simulink model "SWC_OUTP_type"  (R2021b)
settings: Solver=FixedStepDiscrete  StartTime=0.0  StopTime=10.0  FixedStep=0.005  RelTol=1e-3
undefined symbols (not defined in the file): FALSE, TRUE
libraries: outp x1
settings Model: DataDictionary=APPTypes.sldd  Creator=FVT23010  LastModifiedBy=FVT23033
settings DataIOCC: SaveFormat=StructureWithTime
settings OptimizationCC: DefaultParameterBehavior=Inlined  EnhancedBackFolding=on  PassReuseOutputArgsAs=Individual arguments  ZeroExternalMemoryAtStartup=off  ZeroInternalMemoryAtStartup=off  OptimizeBlockOrder=speed  DifferentSizesBufferReuse=on  OptimizationCustomize=off  EfficientTunableParamExpr=on
settings DebuggingCC: ParameterTunabilityLossMsg=error
settings HardwareCC: ProdBitPerPointer=32  ProdBitPerSizeT=32  ProdBitPerPtrDiffT=32  ProdLargestAtomicInteger=Long  ProdLargestAtomicFloat=Double  ProdWordSize=32  ProdLongLongMode=on  ProdHWDeviceType=ARM Compatible->ARM Cortex-M
settings ModelReferenceCC: ModelReferenceNumInstancesAllowed=Single
settings SFSimCC: MATLABDynamicMemAlloc=off
settings RTWCC: Description=AUTOSAR  SystemTargetFile=autosar.tlc  GenCodeOnly=on  TemplateMakefile=ert_default_tmf  PortableWordSizes=on
settings CodeAppCC: ForceParamTrailComments=on  IgnoreCustomStorageClasses=off  OperatorAnnotations=on  SimulinkDataObjDesc=on  SFDataObjDesc=on  InsertBlockDesc=on
settings STFCustomTargetCC: TargetLangStandard=C99 (ISO)  UtilityFuncGeneration=Shared location  MultiwordLength=256  ParMdlRefBuildCompliant=on  CompOptLevelCompliant=on  IncludeMdlTerminateFcn=off  CombineOutputUpdateFcns=on  SuppressErrorStatus=on  ERTCustomFileBanners=on  SupportNonFinite=off  SupportComplex=off  SupportContinuousTime=off  SupportNonInlinedSFcns=off  RemoveResetFunc=on  MATLABClassNameForMDSCustomization=Simulink.SoftwareTarget.ERTCustomization  AutosarCompliant=on  GRTInterface=off  UseToolchainInfoCompliant=on  GenerateSharedConstants=off  LookupTableObjectStructAxisOrder=2,1,3,4,...  LUTObjectStructOrderEvenSpacing=Size,Table,Breakpoints  SystemTargetFile=autosar.tlc
settings ERTTargetCC: TargetLangStandard=C99 (ISO)  UtilityFuncGeneration=Shared location  ConcurrentExecutionCompliant=off  IncludeMdlTerminateFcn=off  SuppressErrorStatus=on  SupportNonFinite=off  SupportComplex=off  ModelStepFunctionPrototypeControlCompliant=off  CPPClassGenCompliant=off  AutosarCompliant=on  GenerateSharedConstants=off  LookupTableObjectStructAxisOrder=2,1,3,4,...  LUTObjectStructOrderEvenSpacing=Size,Table,Breakpoints  GenerateASAP2=on  InlinedParameterPlacement=NonHierarchical  ERTCustomFileTemplate=example_file_process.tlc  ConvertIfToSwitch=off  SuppressUnreachableDefaultCases=off  BooleanTrueId=true_MatlabRTW  BooleanFalseId=false_MatlabRTW

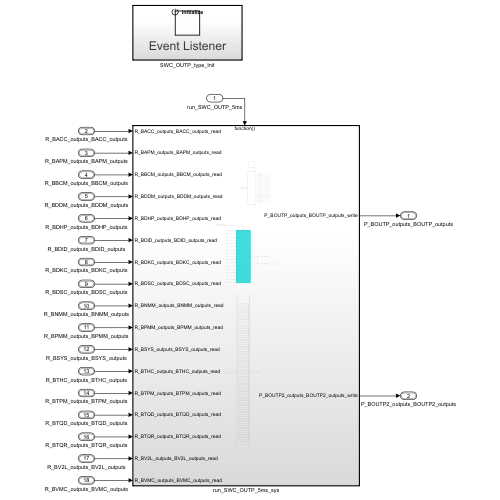
[thumbnail: Simulink's stored preview of the top-level diagram]
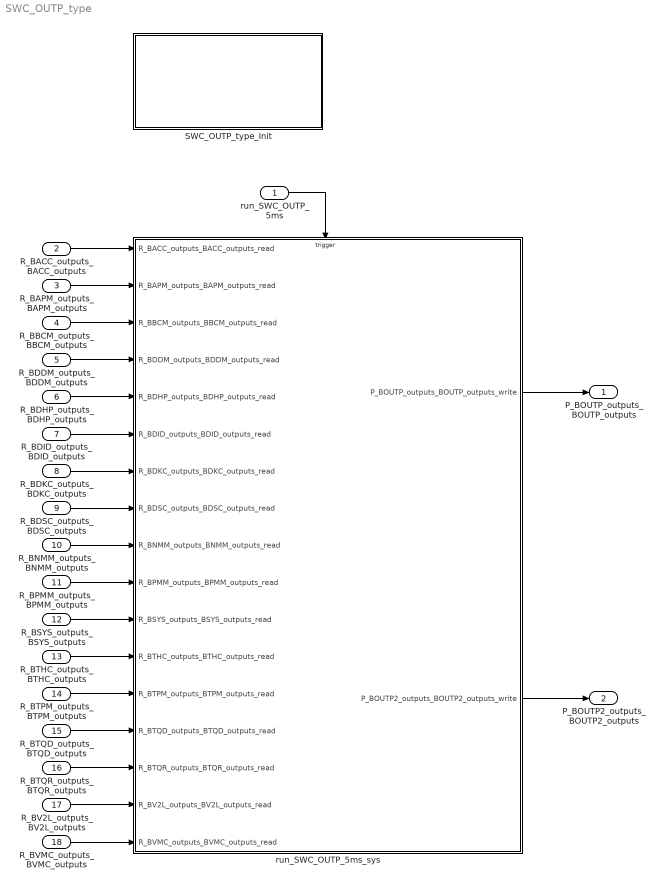
== system SWC_OUTP_type ==
  run_SWC_OUTP_5ms : Inport  SampleTime=0.005  OutputFunctionCall=on
  R_BACC_outputs_BACC_outputs : Inport  Port=2  OutDataTypeStr=Bus: BACC_outputs  PortDimensions=1  BusOutputAsStruct=on
  R_BAPM_outputs_BAPM_outputs : Inport  Port=3  OutDataTypeStr=Bus: BAPM_outputs  PortDimensions=1  BusOutputAsStruct=on
  R_BBCM_outputs_BBCM_outputs : Inport  Port=4  OutDataTypeStr=Bus: BBCM_outputs  PortDimensions=1  BusOutputAsStruct=on
  R_BDDM_outputs_BDDM_outputs : Inport  Port=5  OutDataTypeStr=Bus: BDDM_outputs  PortDimensions=1  BusOutputAsStruct=on
  R_BDHP_outputs_BDHP_outputs : Inport  Port=6  OutDataTypeStr=Bus: BDHP_outputs  PortDimensions=1  BusOutputAsStruct=on
  R_BDID_outputs_BDID_outputs : Inport  Port=7  OutDataTypeStr=Bus: BDID_outputs  PortDimensions=1  BusOutputAsStruct=on
  R_BDKC_outputs_BDKC_outputs : Inport  Port=8  OutDataTypeStr=Bus: BDKC_outputs  PortDimensions=1  BusOutputAsStruct=on
  R_BDSC_outputs_BDSC_outputs : Inport  Port=9  OutDataTypeStr=Bus: BDSC_outputs  PortDimensions=1  BusOutputAsStruct=on
  R_BNMM_outputs_BNMM_outputs : Inport  Port=10  OutDataTypeStr=Bus: BNMM_outputs  PortDimensions=1  BusOutputAsStruct=on
  R_BPMM_outputs_BPMM_outputs : Inport  Port=11  OutDataTypeStr=Bus: BPMM_outputs  PortDimensions=1  BusOutputAsStruct=on
  R_BSYS_outputs_BSYS_outputs : Inport  Port=12  OutDataTypeStr=Bus: BSYS_outputs  PortDimensions=1  BusOutputAsStruct=on
  R_BTHC_outputs_BTHC_outputs : Inport  Port=13  OutDataTypeStr=Bus: BTHC_outputs  PortDimensions=1  BusOutputAsStruct=on
  R_BTPM_outputs_BTPM_outputs : Inport  Port=14  OutDataTypeStr=Bus: BTPM_outputs  PortDimensions=1  BusOutputAsStruct=on
  R_BTQD_outputs_BTQD_outputs : Inport  Port=15  OutDataTypeStr=Bus: BTQD_outputs  PortDimensions=1  BusOutputAsStruct=on
  R_BTQR_outputs_BTQR_outputs : Inport  Port=16  OutDataTypeStr=Bus: BTQR_outputs  PortDimensions=1  BusOutputAsStruct=on
  R_BV2L_outputs_BV2L_outputs : Inport  Port=17  OutDataTypeStr=Bus: BV2L_outputs  PortDimensions=1  BusOutputAsStruct=on
  R_BVMC_outputs_BVMC_outputs : Inport  Port=18  OutDataTypeStr=Bus: BVMC_outputs  PortDimensions=1  BusOutputAsStruct=on
  SWC_OUTP_type_Init : Subsystem
  run_SWC_OUTP_5ms_sys : Subsystem
  P_BOUTP_outputs_BOUTP_outputs : Outport  OutDataTypeStr=Bus: BOUTP_outputs  PortDimensions=1  BusOutputAsStruct=on
  P_BOUTP2_outputs_BOUTP2_outputs : Outport  Port=2  OutDataTypeStr=Bus: BOUTP2_outputs  PortDimensions=1  BusOutputAsStruct=on
  wires:
  R_BACC_outputs_BACC_outputs/1 -> run_SWC_OUTP_5ms_sys/1(R_BACC_outputs_BACC_outputs_read)
  R_BAPM_outputs_BAPM_outputs/1 -> run_SWC_OUTP_5ms_sys/2(R_BAPM_outputs_BAPM_outputs_read)
  R_BBCM_outputs_BBCM_outputs/1 -> run_SWC_OUTP_5ms_sys/3(R_BBCM_outputs_BBCM_outputs_read)
  R_BDDM_outputs_BDDM_outputs/1 -> run_SWC_OUTP_5ms_sys/4(R_BDDM_outputs_BDDM_outputs_read)
  R_BDHP_outputs_BDHP_outputs/1 -> run_SWC_OUTP_5ms_sys/5(R_BDHP_outputs_BDHP_outputs_read)
  R_BDID_outputs_BDID_outputs/1 -> run_SWC_OUTP_5ms_sys/6(R_BDID_outputs_BDID_outputs_read)
  R_BDKC_outputs_BDKC_outputs/1 -> run_SWC_OUTP_5ms_sys/7(R_BDKC_outputs_BDKC_outputs_read)
  R_BDSC_outputs_BDSC_outputs/1 -> run_SWC_OUTP_5ms_sys/8(R_BDSC_outputs_BDSC_outputs_read)
  R_BNMM_outputs_BNMM_outputs/1 -> run_SWC_OUTP_5ms_sys/9(R_BNMM_outputs_BNMM_outputs_read)
  R_BPMM_outputs_BPMM_outputs/1 -> run_SWC_OUTP_5ms_sys/10(R_BPMM_outputs_BPMM_outputs_read)
  R_BSYS_outputs_BSYS_outputs/1 -> run_SWC_OUTP_5ms_sys/11(R_BSYS_outputs_BSYS_outputs_read)
  R_BTHC_outputs_BTHC_outputs/1 -> run_SWC_OUTP_5ms_sys/12(R_BTHC_outputs_BTHC_outputs_read)
  R_BTPM_outputs_BTPM_outputs/1 -> run_SWC_OUTP_5ms_sys/13(R_BTPM_outputs_BTPM_outputs_read)
  R_BTQD_outputs_BTQD_outputs/1 -> run_SWC_OUTP_5ms_sys/14(R_BTQD_outputs_BTQD_outputs_read)
  R_BTQR_outputs_BTQR_outputs/1 -> run_SWC_OUTP_5ms_sys/15(R_BTQR_outputs_BTQR_outputs_read)
  R_BV2L_outputs_BV2L_outputs/1 -> run_SWC_OUTP_5ms_sys/16(R_BV2L_outputs_BV2L_outputs_read)
  R_BVMC_outputs_BVMC_outputs/1 -> run_SWC_OUTP_5ms_sys/17(R_BVMC_outputs_BVMC_outputs_read)
  run_SWC_OUTP_5ms_sys/1(P_BOUTP_outputs_BOUTP_outputs_write) -> P_BOUTP_outputs_BOUTP_outputs/1
  run_SWC_OUTP_5ms_sys/2(P_BOUTP2_outputs_BOUTP2_outputs_write) -> P_BOUTP2_outputs_BOUTP2_outputs/1
  run_SWC_OUTP_5ms/1 -> run_SWC_OUTP_5ms_sys/Trigger

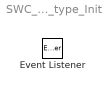
== system SWC_OUTP_type/SWC_OUTP_type_Init ==
  Event Listener : EventListener  EventName=reset

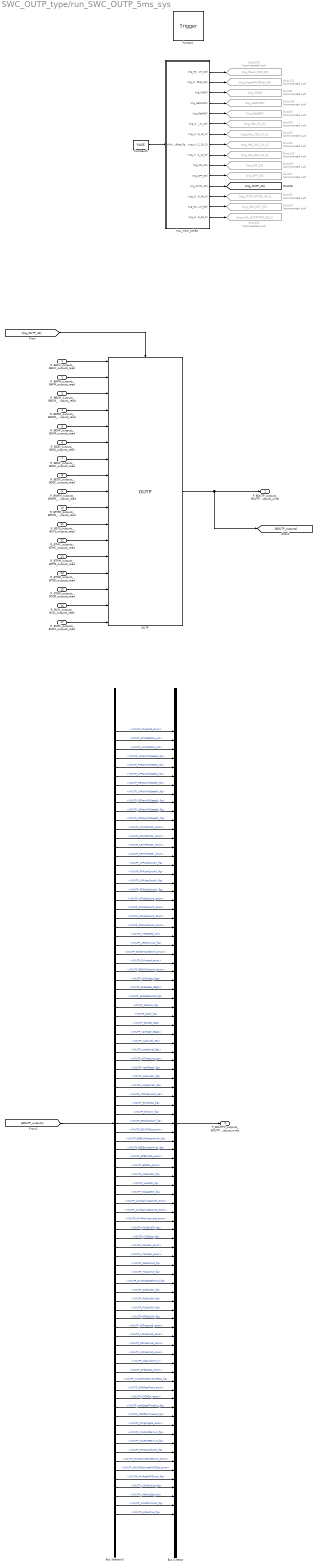
== system SWC_OUTP_type/run_SWC_OUTP_5ms_sys ==
  R_BACC_outputs_BACC_outputs_read : Inport
  R_BAPM_outputs_BAPM_outputs_read : Inport  Port=2
  R_BBCM_outputs_BBCM_outputs_read : Inport  Port=3
  R_BDDM_outputs_BDDM_outputs_read : Inport  Port=4
  R_BDHP_outputs_BDHP_outputs_read : Inport  Port=5
  R_BDID_outputs_BDID_outputs_read : Inport  Port=6
  R_BDKC_outputs_BDKC_outputs_read : Inport  Port=7
  R_BDSC_outputs_BDSC_outputs_read : Inport  Port=8
  R_BNMM_outputs_BNMM_outputs_read : Inport  Port=9
  R_BPMM_outputs_BPMM_outputs_read : Inport  Port=10
  R_BSYS_outputs_BSYS_outputs_read : Inport  Port=11
  R_BTHC_outputs_BTHC_outputs_read : Inport  Port=12
  R_BTPM_outputs_BTPM_outputs_read : Inport  Port=13
  R_BTQD_outputs_BTQD_outputs_read : Inport  Port=14
  R_BTQR_outputs_BTQR_outputs_read : Inport  Port=15
  R_BV2L_outputs_BV2L_outputs_read : Inport  Port=16
  R_BVMC_outputs_BVMC_outputs_read : Inport  Port=17
  function : TriggerPort  TriggerType=function-call  VariantControl=(inherit)  SampleTimeType=periodic  SampleTime=-1
  Bus Creator : BusCreator  Inputs=89  OutDataTypeStr=Bus: BOUTP2_outputs  NonVirtualBus=on
  Bus Selector3 : BusSelector  OutputSignals=VOUTP_PowerSta_enum,VOUTP_BrkPedalPos_pct,VOUTP_ActAPSPosn_pct,VOUTP_LFRawWhlSpeed_kph,VOUTP_RFRawWhlSpeed_kph,VOUTP_LRRawWhlSpeed_kph,VOUTP_RRRawWhlSpeed_kph,VOUTP_LFRawWhlSpeedV_flg,VOUTP_RFRawWhlSpeedV_flg,VOUTP_LRRawWhlSpeedV_flg,VOUTP_RRRawWhlSpeedV_flg,VOUTP_LFWhlRotDir_enum,VOUTP_RFWhlRotDir_enum,VOUTP_LRWhlRotDir_enum,VOUTP_RRWhlRotDir_enum,VOUTP_LFPulseCountV_flg,VOUTP_RFPulseCountV_flg,VOUTP_LRPulseCountV_flg,VOUTP_RRPulseCountV_flg,VOUTP_LFPulseCount_enum,VOUTP_RFPulseCount_enum,VOUTP_LRPulseCount_enum,VOUTP_RRPulseCount_enum,VOUTP_VehSpeed_kph,VOUTP_APSCtrlAvail_flg,VOUTP_ShifterHandleCmd_enum,VOUTP_DriIntend_enum,VOUTP_EPSAOIControl_enum,VOUTP_SASAngle_Deg,VOUTP_SASSpeed_degps,VOUTP_SASSpeedValid_flg,VOUTP_SASCAL_flg,VOUTP_SASV_flg,VOUTP_GRADE_Deg,VOUTP_YawRate_degps,VOUTP_LatAccel_Gps,VOUTP_LongAccel_Gps,VOUTP_MCPressure_bar,VOUTP_YawRateV_flg,VOUTP_LatAccelV_flg,VOUTP_LongAccelV_flg,VOUTP_MCPressureV_bar,VOUTP_BrkSwSta_flg,VOUTP_BrkSwV_flg,VOUTP_ESCStandstill_flg,VOUTP_ESCAPSSta_enum,VOUTP_EPBExtReleaseAvail_flg,VOUTP_EPBExtApplyAvail_flg,VOUTP_EPBErrSta_enum,VOUTP_EPBSta_enum,VOUTP_AllDoorSW_flg,VOUTP_HoodSW_flg,VOUTP_TailgateSW_flg,VOUTP_AVMparkingcancel_enum,VOUTP_AVMparkingexcute_enum,VOUTP_AVMParkingmode_enum,VOUTP_AVMErrSTA_flg,VOUTP_IVIStatus_flg,VOUTP_CAASSw_enum,VOUTP_IVIScreen_enum,VOUTP_ABSActive_flg,VOUTP_TCSActive_flg,VOUTP_DriverSeatBeltCmd_flg,VOUTP_DrDoorSW_flg,VOUTP_PsDoorSW_flg,VOUTP_RLDoorSW_flg,VOUTP_RRDoorSW_flg,VOUTP_RFPressIndi_enum,VOUTP_LFPressIndi_enum,VOUTP_RRPressIndi_enum,VOUTP_LRPressIndi_enum,VOUTP_sigAmbAirT_C,VOUTP_DrSeatSta_enum,VOUTP_IVIUserTakeOverAPSSta_flg,VOUTP_ShiftGearPosn_enum,VOUTP_FSOffSw_enum,VOUTP_VehSpeedTimeOut_flg,VOUTP_FSOffSwTimeOut_flg,VOUTP_ChrgPlugSta_enum,VOUTP_VCURAPSErrLv2_flg,VOUTP_VCURAPSErrLv3_flg,VOUTP_PUIDLowPower_flg,VOUTP_DKCParkingModeCmd_enum,VOUTP_DKCPDkeyAreaRAPSSta_enum,VOUTP_PwrReqRAPSAvail_flg,VOUTP_CAASActive_flg,VOUTP_VehActSpd_kph,VOUTP_CAASCtrlAvail_flg,VOUTP_APSActive_flg
  Constant5 : Constant  Value=FALSE
  Goto100 : Goto  Commented=on  GotoTag=trig_Read_NVM_00
  Goto101 : Goto  Commented=on  GotoTag=trig_HAL_OUTAFTER_50_1
  Goto102 : Goto  Commented=on  GotoTag=trig_ReadIMUOffset_00
  Goto106 : Goto  Commented=on  GotoTag=trig_GetNMID
  Goto119 : Goto  Commented=on  GotoTag=trig_HAL_DKC_10_3
  Goto90 : Goto  Commented=on  GotoTag=trig_GetDID
  Goto91 : Goto  Commented=on  GotoTag=trig_WDG
  Goto92 : Goto  Commented=on  GotoTag=trig_HAL_DKC_10_2
  Goto93 : Goto  Commented=on  GotoTag=trig_HAL_CDD_10_1
  Goto94 : Goto  Commented=on  GotoTag=trig_HAL_OUT_50
  Goto95 : Goto  Commented=on  GotoTag=trig_OUTP_AFTER_40_1
  Goto97 : Goto  Commented=on  GotoTag=trig_APP_30
  Goto98 : Goto  Commented=on  GotoTag=trig_INP_20
  Goto99 : Goto  Commented=on  GotoTag=trig_HAL_IN_10
  OUTP : outp/OUTP  SystemSampleTime=-1  VariantActivationTime=update diagram  Latency=0  AutoFrameSizeCalculation=off
  hcu_main_sched : Stateflow chart  TreatAsAtomicUnit=on
  P_BOUTP_outputs_BOUTP_outputs_write : Outport
  P_BOUTP2_outputs_BOUTP2_outputs_write : Outport  Port=2
  wires:
  hcu_main_sched/2(trig_ReadIMUOffset_00()) -> Goto102/1
  hcu_main_sched/5(trig_GetDID()) -> Goto90/1
  hcu_main_sched/15(trig_HAL_OUTAFTER_50_1()) -> Goto101/1
  hcu_main_sched/12(trig_OUTP_40()) -> [trig_OUTP_40]
  hcu_main_sched/3(trig_WDG()) -> Goto91/1
  hcu_main_sched/6(trig_HAL_IN_10()) -> Goto99/1
  hcu_main_sched/4(trig_GetNMID()) -> Goto106/1
  hcu_main_sched/14(trig_HAL_OUT_50()) -> Goto94/1
  hcu_main_sched/9(trig_HAL_DKC_10_3()) -> Goto119/1
  hcu_main_sched/1(trig_Read_NVM_00()) -> Goto100/1
  Constant5/1 -> hcu_main_sched/1(VHAL_FusionSchedReq_flg)
  hcu_main_sched/13(trig_OUTP_AFTER_40_1()) -> Goto95/1
  hcu_main_sched/11(trig_APP_30()) -> Goto97/1
  hcu_main_sched/8(trig_HAL_DKC_10_2()) -> Goto92/1
  hcu_main_sched/10(trig_INP_20()) -> Goto98/1
  hcu_main_sched/7(trig_HAL_CDD_10_1()) -> Goto93/1
  OUTP/1 -> P_BOUTP_outputs_BOUTP_outputs_write/1, [BOUTP_outputs]
  [trig_OUTP_40] -> OUTP/Trigger
  R_BPMM_outputs_BPMM_outputs_read/1 -> OUTP/10
  R_BNMM_outputs_BNMM_outputs_read/1 -> OUTP/9
  R_BSYS_outputs_BSYS_outputs_read/1 -> OUTP/11
  R_BDSC_outputs_BDSC_outputs_read/1 -> OUTP/8
  R_BTHC_outputs_BTHC_outputs_read/1 -> OUTP/12
  R_BDKC_outputs_BDKC_outputs_read/1 -> OUTP/7
  R_BTPM_outputs_BTPM_outputs_read/1 -> OUTP/13
  R_BDID_outputs_BDID_outputs_read/1 -> OUTP/6
  R_BTQD_outputs_BTQD_outputs_read/1 -> OUTP/14
  R_BDHP_outputs_BDHP_outputs_read/1 -> OUTP/5
  R_BTQR_outputs_BTQR_outputs_read/1 -> OUTP/15
  R_BDDM_outputs_BDDM_outputs_read/1 -> OUTP/4
  R_BV2L_outputs_BV2L_outputs_read/1 -> OUTP/16
  R_BBCM_outputs_BBCM_outputs_read/1 -> OUTP/3
  R_BVMC_outputs_BVMC_outputs_read/1 -> OUTP/17
  R_BAPM_outputs_BAPM_outputs_read/1 -> OUTP/2
  R_BACC_outputs_BACC_outputs_read/1 -> OUTP/1
  Bus Selector3/75 -> Bus Creator/75  "<VOUTP_ShiftGearPosn_enum>"
  Bus Creator/1 -> P_BOUTP2_outputs_BOUTP2_outputs_write/1
  Bus Selector3/79 -> Bus Creator/79  "<VOUTP_ChrgPlugSta_enum>"
  Bus Selector3/61 -> Bus Creator/61  "<VOUTP_ABSActive_flg>"
  Bus Selector3/78 -> Bus Creator/78  "<VOUTP_FSOffSwTimeOut_flg>"
  Bus Selector3/54 -> Bus Creator/54  "<VOUTP_AVMparkingcancel_enum>"
  Bus Selector3/69 -> Bus Creator/69  "<VOUTP_LFPressIndi_enum>"
  Bus Selector3/30 -> Bus Creator/30  "<VOUTP_SASSpeed_degps>"
  Bus Selector3/77 -> Bus Creator/77  "<VOUTP_VehSpeedTimeOut_flg>"
  Bus Selector3/70 -> Bus Creator/70  "<VOUTP_RRPressIndi_enum>"
  Bus Selector3/1 -> Bus Creator/1  "<VOUTP_PowerSta_enum>"
  Bus Selector3/72 -> Bus Creator/72  "<VOUTP_sigAmbAirT_C>"
  Bus Selector3/21 -> Bus Creator/21  "<VOUTP_RFPulseCount_enum>"
  Bus Selector3/46 -> Bus Creator/46  "<VOUTP_ESCAPSSta_enum>"
  Bus Selector3/71 -> Bus Creator/71  "<VOUTP_LRPressIndi_enum>"
  Bus Selector3/18 -> Bus Creator/18  "<VOUTP_LRPulseCountV_flg>"
  Bus Selector3/65 -> Bus Creator/65  "<VOUTP_PsDoorSW_flg>"
  Bus Selector3/68 -> Bus Creator/68  "<VOUTP_RFPressIndi_enum>"
  Bus Selector3/73 -> Bus Creator/73  "<VOUTP_DrSeatSta_enum>"
  Bus Selector3/76 -> Bus Creator/76  "<VOUTP_FSOffSw_enum>"
  Bus Selector3/74 -> Bus Creator/74  "<VOUTP_IVIUserTakeOverAPSSta_flg>"
  Bus Selector3/22 -> Bus Creator/22  "<VOUTP_LRPulseCount_enum>"
  Bus Selector3/16 -> Bus Creator/16  "<VOUTP_LFPulseCountV_flg>"
  Bus Selector3/41 -> Bus Creator/41  "<VOUTP_LongAccelV_flg>"
  Bus Selector3/67 -> Bus Creator/67  "<VOUTP_RRDoorSW_flg>"
  Bus Selector3/62 -> Bus Creator/62  "<VOUTP_TCSActive_flg>"
  Bus Selector3/38 -> Bus Creator/38  "<VOUTP_MCPressure_bar>"
  Bus Selector3/56 -> Bus Creator/56  "<VOUTP_AVMParkingmode_enum>"
  Bus Selector3/58 -> Bus Creator/58  "<VOUTP_IVIStatus_flg>"
  Bus Selector3/55 -> Bus Creator/55  "<VOUTP_AVMparkingexcute_enum>"
  Bus Selector3/4 -> Bus Creator/4  "<VOUTP_LFRawWhlSpeed_kph>"
  Bus Selector3/57 -> Bus Creator/57  "<VOUTP_AVMErrSTA_flg>"
  Bus Selector3/59 -> Bus Creator/59  "<VOUTP_CAASSw_enum>"
  Bus Selector3/34 -> Bus Creator/34  "<VOUTP_GRADE_Deg>"
  Bus Selector3/40 -> Bus Creator/40  "<VOUTP_LatAccelV_flg>"
  Bus Selector3/47 -> Bus Creator/47  "<VOUTP_EPBExtReleaseAvail_flg>"
  Bus Selector3/50 -> Bus Creator/50  "<VOUTP_EPBSta_enum>"
  Bus Selector3/48 -> Bus Creator/48  "<VOUTP_EPBExtApplyAvail_flg>"
  Bus Selector3/49 -> Bus Creator/49  "<VOUTP_EPBErrSta_enum>"
  Bus Selector3/52 -> Bus Creator/52  "<VOUTP_HoodSW_flg>"
  Bus Selector3/2 -> Bus Creator/2  "<VOUTP_BrkPedalPos_pct>"
  Bus Selector3/66 -> Bus Creator/66  "<VOUTP_RLDoorSW_flg>"
  Bus Selector3/32 -> Bus Creator/32  "<VOUTP_SASCAL_flg>"
  Bus Selector3/53 -> Bus Creator/53  "<VOUTP_TailgateSW_flg>"
  Bus Selector3/26 -> Bus Creator/26  "<VOUTP_ShifterHandleCmd_enum>"
  Bus Selector3/51 -> Bus Creator/51  "<VOUTP_AllDoorSW_flg>"
  Bus Selector3/31 -> Bus Creator/31  "<VOUTP_SASSpeedValid_flg>"
  Bus Selector3/24 -> Bus Creator/24  "<VOUTP_VehSpeed_kph>"
  Bus Selector3/9 -> Bus Creator/9  "<VOUTP_RFRawWhlSpeedV_flg>"
  Bus Selector3/64 -> Bus Creator/64  "<VOUTP_DrDoorSW_flg>"
  Bus Selector3/39 -> Bus Creator/39  "<VOUTP_YawRateV_flg>"
  Bus Selector3/42 -> Bus Creator/42  "<VOUTP_MCPressureV_bar>"
  Bus Selector3/28 -> Bus Creator/28  "<VOUTP_EPSAOIControl_enum>"
  Bus Selector3/60 -> Bus Creator/60  "<VOUTP_IVIScreen_enum>"
  Bus Selector3/36 -> Bus Creator/36  "<VOUTP_LatAccel_Gps>"
  Bus Selector3/33 -> Bus Creator/33  "<VOUTP_SASV_flg>"
  Bus Selector3/37 -> Bus Creator/37  "<VOUTP_LongAccel_Gps>"
  Bus Selector3/35 -> Bus Creator/35  "<VOUTP_YawRate_degps>"
  Bus Selector3/29 -> Bus Creator/29  "<VOUTP_SASAngle_Deg>"
  Bus Selector3/45 -> Bus Creator/45  "<VOUTP_ESCStandstill_flg>"
  Bus Selector3/43 -> Bus Creator/43  "<VOUTP_BrkSwSta_flg>"
  Bus Selector3/44 -> Bus Creator/44  "<VOUTP_BrkSwV_flg>"
  Bus Selector3/63 -> Bus Creator/63  "<VOUTP_DriverSeatBeltCmd_flg>"
  Bus Selector3/12 -> Bus Creator/12  "<VOUTP_LFWhlRotDir_enum>"
  Bus Selector3/14 -> Bus Creator/14  "<VOUTP_LRWhlRotDir_enum>"
  Bus Selector3/17 -> Bus Creator/17  "<VOUTP_RFPulseCountV_flg>"
  Bus Selector3/25 -> Bus Creator/25  "<VOUTP_APSCtrlAvail_flg>"
  Bus Selector3/15 -> Bus Creator/15  "<VOUTP_RRWhlRotDir_enum>"
  Bus Selector3/8 -> Bus Creator/8  "<VOUTP_LFRawWhlSpeedV_flg>"
  Bus Selector3/27 -> Bus Creator/27  "<VOUTP_DriIntend_enum>"
  Bus Selector3/10 -> Bus Creator/10  "<VOUTP_LRRawWhlSpeedV_flg>"
  Bus Selector3/13 -> Bus Creator/13  "<VOUTP_RFWhlRotDir_enum>"
  Bus Selector3/11 -> Bus Creator/11  "<VOUTP_RRRawWhlSpeedV_flg>"
  Bus Selector3/23 -> Bus Creator/23  "<VOUTP_RRPulseCount_enum>"
  Bus Selector3/5 -> Bus Creator/5  "<VOUTP_RFRawWhlSpeed_kph>"
  Bus Selector3/3 -> Bus Creator/3  "<VOUTP_ActAPSPosn_pct>"
  Bus Selector3/6 -> Bus Creator/6  "<VOUTP_LRRawWhlSpeed_kph>"
  [BOUTP_outputs] -> Bus Selector3/1
  Bus Selector3/20 -> Bus Creator/20  "<VOUTP_LFPulseCount_enum>"
  Bus Selector3/7 -> Bus Creator/7  "<VOUTP_RRRawWhlSpeed_kph>"
  Bus Selector3/19 -> Bus Creator/19  "<VOUTP_RRPulseCountV_flg>"
  Bus Selector3/80 -> Bus Creator/80  "<VOUTP_VCURAPSErrLv2_flg>"
  Bus Selector3/81 -> Bus Creator/81  "<VOUTP_VCURAPSErrLv3_flg>"
  Bus Selector3/82 -> Bus Creator/82  "<VOUTP_PUIDLowPower_flg>"
  Bus Selector3/83 -> Bus Creator/83  "<VOUTP_DKCParkingModeCmd_enum>"
  Bus Selector3/84 -> Bus Creator/84  "<VOUTP_DKCPDkeyAreaRAPSSta_enum>"
  Bus Selector3/85 -> Bus Creator/85  "<VOUTP_PwrReqRAPSAvail_flg>"
  Bus Selector3/86 -> Bus Creator/86  "<VOUTP_CAASActive_flg>"
  Bus Selector3/87 -> Bus Creator/87  "<VOUTP_VehActSpd_kph>"
  Bus Selector3/88 -> Bus Creator/88  "<VOUTP_CAASCtrlAvail_flg>"
  Bus Selector3/89 -> Bus Creator/89  "<VOUTP_APSActive_flg>"

== stateflow chart SWC_OUTP_type/run_SWC_OUTP_5ms_sys/hcu_main_sched ==
  state Main_Scheduler
    (default) -> (junction 31) : {
        |   Sys_Init_done = FALSE;
        |   trig_Read_NVM_00;
        |   trig_ReadIMUOffset_00;
        | }
    Main_Scheduler -> (junction 31) : {Sys_Init_done = TRUE;}
    (junction 31) -> (junction 34) [order 1] : [
        |    Sys_Init_done &&...
        |    !VHAL_FusionSchedReq_flg
        | ]
    (junction 31) -> (junction 38) [order 2]
    (junction 34) -> (junction 36) : {
        |     trig_WDG;
        |     trig_GetNMID;
        |     trig_GetDID;
        |     trig_HAL_IN_10;
        |     trig_HAL_CDD_10_1;
        |     trig_HAL_DKC_10_2;
        |     trig_HAL_DKC_10_3;
        |     trig_INP_20;
        |     trig_APP_30;
        |     trig_OUTP_40;
        |     trig_OUTP_AFTER_40_1;
        |     trig_HAL_OUT_50;
        |     trig_HAL_OUTAFTER_50_1;
        |    }
    (junction 36) -> (junction 38)
  (default) -> Main_Scheduler
  data: VHAL_FusionSchedReq_flg input; Sys_Init_done local double; FALSE parameter; TRUE parameter
  events: trig_Read_NVM_00 output FUNCTION_CALL_EVENT; trig_ReadIMUOffset_00 output FUNCTION_CALL_EVENT; trig_WDG output FUNCTION_CALL_EVENT; trig_GetNMID output FUNCTION_CALL_EVENT; trig_GetDID output FUNCTION_CALL_EVENT; trig_HAL_IN_10 output FUNCTION_CALL_EVENT; trig_HAL_CDD_10_1 output FUNCTION_CALL_EVENT; trig_HAL_DKC_10_2 output FUNCTION_CALL_EVENT; trig_HAL_DKC_10_3 output FUNCTION_CALL_EVENT; trig_INP_20 output FUNCTION_CALL_EVENT; trig_APP_30 output FUNCTION_CALL_EVENT; trig_OUTP_40 output FUNCTION_CALL_EVENT; trig_OUTP_AFTER_40_1 output FUNCTION_CALL_EVENT; trig_HAL_OUT_50 output FUNCTION_CALL_EVENT; trig_HAL_OUTAFTER_50_1 output FUNCTION_CALL_EVENT
